simulink model "chap5_9sim"  (Simulink 7.7)
settings: Solver=ode45  StartTime=0.0  StopTime=20  FixedStep=0.001  RelTol=1e-3
libraries: simulink x1
settings Model: Creator=hp  LastModifiedBy=ljk  ExtModeTrigMode=oneshot  ExtModeArmWhenConnect=off
settings DataIOCC: LimitDataPoints=off  SignalLoggingName=sigsOut
settings OptimizationCC: BooleanDataType=off  InitFltsAndDblsToZero=on
settings DebuggingCC: SaveWithParameterizedLinksMsg=none  SignalResolutionControl=TryResolveAllWithWarning  SolverPrmCheckMsg=none  MultiTaskDSMMsg=warning  MultiTaskCondExecSysMsg=none  StrictBusMsg=None
settings HardwareCC: TargetUnknown=on
settings RTWCC: IncludeERTFirstTime=on
settings GRTTargetCC: TargetFcnLib=ansi_tfl_tmw.mat

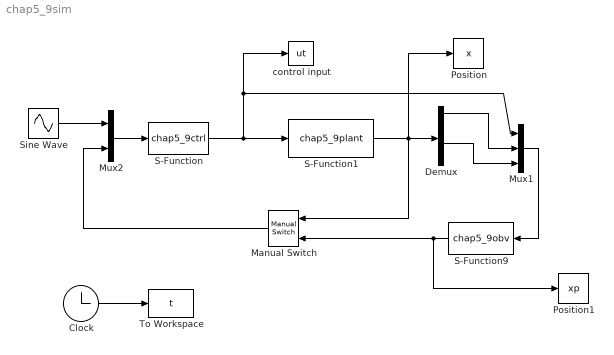
== system chap5_9sim ==
  Clock : Clock
      settings: Decimation=10
  Demux : Demux
  Manual Switch : simulink/Signal Routing/Manual Switch  SystemSampleTime=-1  sw=0  action=0  varsize=off
  Mux1 : Mux  Inputs=3
  Mux2 : Mux  Inputs=2
  Position : ToWorkspace  VariableName=x  SampleTime=-1  SaveFormat=Array
  Position1 : ToWorkspace  VariableName=xp  SampleTime=-1  SaveFormat=Array
  S-Function : S-Function  FunctionName=chap5_9ctrl  EnableBusSupport=off
  S-Function1 : S-Function  FunctionName=chap5_9plant  EnableBusSupport=off
  S-Function9 : S-Function  FunctionName=chap5_9obv  EnableBusSupport=off
  Sine Wave : Sin  SampleTime=0
  To Workspace : ToWorkspace  VariableName=t  SampleTime=-1  SaveFormat=Array
  control input : ToWorkspace  VariableName=ut  SampleTime=-1  SaveFormat=Array
  wires:
  S-Function/1 -> S-Function1/1, control input/1, Mux1/1
  Clock/1 -> To Workspace/1
  S-Function1/1 -> Demux/1, Position/1, Manual Switch/1
  Demux/1 -> Mux1/2
  Demux/3 -> Mux1/3
  Mux1/1 -> S-Function9/1
  Mux2/1 -> S-Function/1
  Sine Wave/1 -> Mux2/1
  S-Function9/1 -> Position1/1, Manual Switch/2
  Manual Switch/1 -> Mux2/2
